simulink model "Battery_ECM"  (R2022b)
settings: Solver=VariableStepAuto  StartTime=0.0  StopTime=30000  RelTol=1e-3
undefined symbols (not defined in the file): C1, C2, eta_charge, eta_discharge, Q_C, R0, R1, R2, SoC0, Ts
settings Model: Creator=Hadi  LastModifiedBy=Hadi

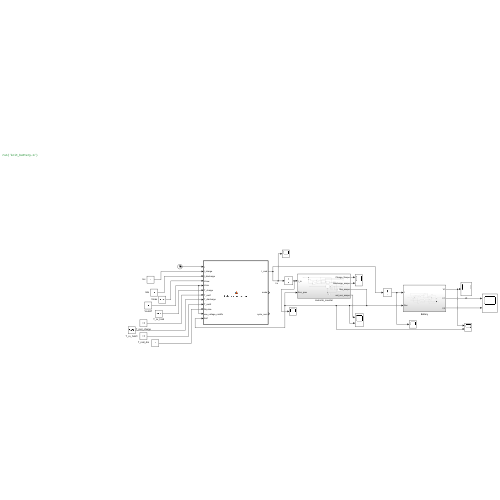
[thumbnail: Simulink's stored preview of the top-level diagram]
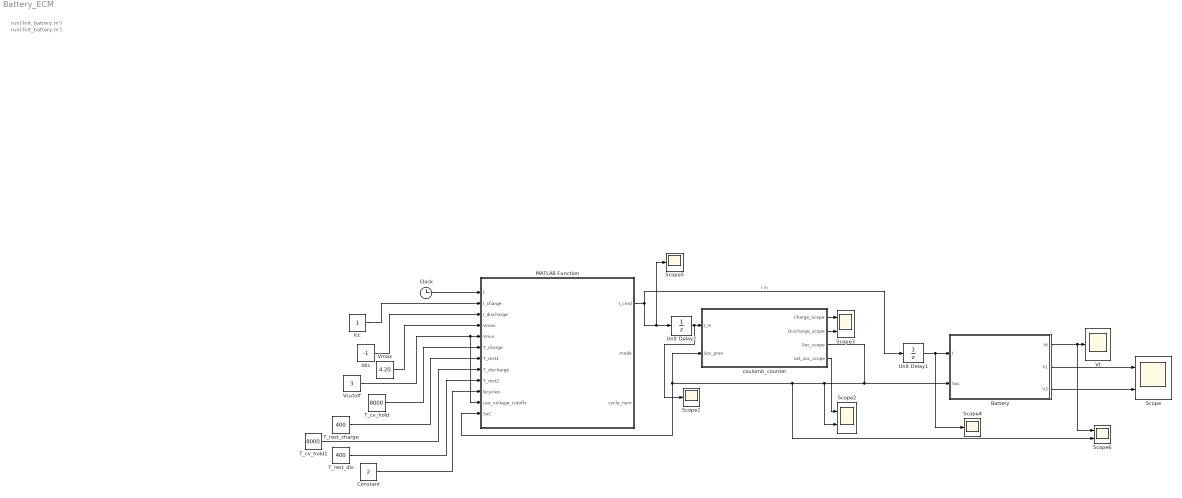
== system Battery_ECM ==
  note: run('init_battery.m')
  note: run('init_battery.m')
  Battery : Subsystem
  Clock : Clock
  Constant : Constant  Value=2
  Icc : Constant
  Idis : Constant  Value=-1
  MATLAB Function : MATLAB Function  TreatAsAtomicUnit=on
  Scope{,2..3,6} (4 alike) : Scope  NumInputPorts=2
  Scope1 : Scope
  Scope4 : Scope
  Scope5 : Scope
  T_cv_hold : Constant  Value=8000
  T_cv_hold1 : Constant  Value=8000
  T_rest_charge : Constant  Value=400
  T_rest_dis : Constant  Value=400
  Unit Delay1 : UnitDelay  SampleTime=0.05  HasFrameUpgradeWarning=on
  Unit Delay2 : UnitDelay  SampleTime=0.05  HasFrameUpgradeWarning=on
  Vcutoff : Constant  Value=3
  Vmax : Constant  Value=4.20
  Vt : Scope
  coulomb_counter : Subsystem
  wires:
  MATLAB Function/1(I_cmd) -> Scope5/1, Unit Delay2/1, Unit Delay1/1  "I in"
  Unit Delay1/1 -> Scope4/1, Battery/1(I)
  coulomb_counter/1(Charge_Scope) -> Scope3/1
  Unit Delay2/1 -> Scope1/1, coulomb_counter/1(I_In)
  coulomb_counter/4(sat_soc_scope) -> Scope2/1
  coulomb_counter/2(Discharge_scope) -> Scope3/2
  coulomb_counter/3(Soc_scope) -> Scope6/2, MATLAB Function/12(SoC), coulomb_counter/2(Soc_prev), Scope2/2, Battery/2(Soc)
  Battery/3(V2) -> Scope/2
  Battery/2(V1) -> Scope/1
  Battery/1(Vt) -> Scope6/1, Vt/1
  Clock/1 -> MATLAB Function/1(t)
  Vmax/1 -> MATLAB Function/4(Vmax)
  Vcutoff/1 -> MATLAB Function/5(Vmin), MATLAB Function/11(use_voltage_cutoffs)
  T_rest_charge/1 -> MATLAB Function/7(T_rest1)
  T_rest_dis/1 -> MATLAB Function/9(T_rest2)
  Icc/1 -> MATLAB Function/2(I_charge)
  Idis/1 -> MATLAB Function/3(I_discharge)
  T_cv_hold/1 -> MATLAB Function/6(T_charge)
  Constant/1 -> MATLAB Function/10(Ncycles)
  T_cv_hold1/1 -> MATLAB Function/8(T_discharge)

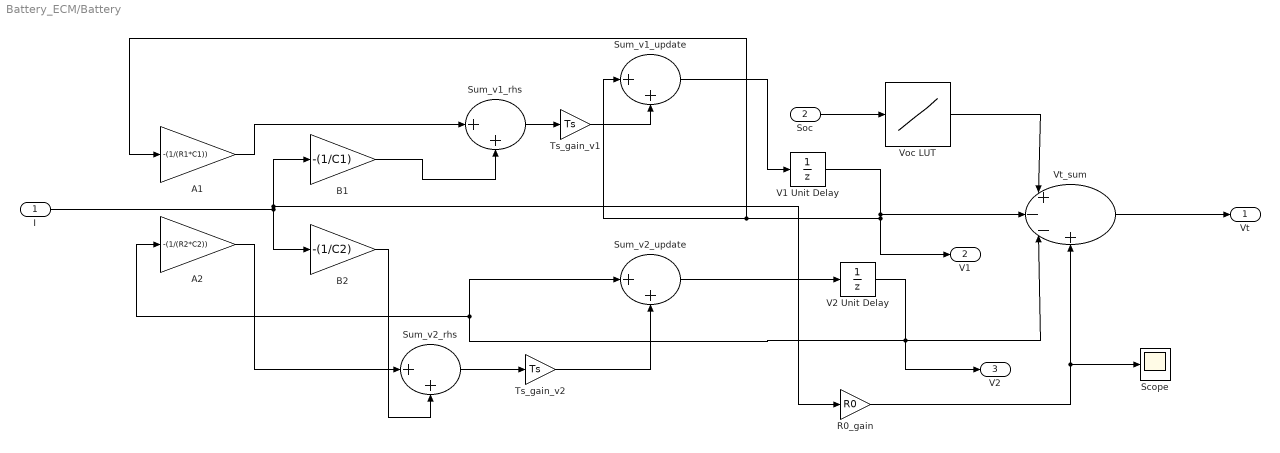
== system Battery_ECM/Battery ==
  I : Inport
  Soc : Inport  Port=2
  A1 : Gain  Gain=-(1/(R1*C1))
  A2 : Gain  Gain=-(1/(R2*C2))
  B1 : Gain  Gain=-(1/C1)
  B2 : Gain  Gain=-(1/C2)
  R0_gain : Gain  Gain=R0
  Scope : Scope
  Sum_v1_rhs : Sum  Inputs=|++
  Sum_v1_update : Sum  Inputs=|++
  Sum_v2_rhs : Sum  Inputs=|++
  Sum_v2_update : Sum  Inputs=|++
  Ts_gain_v1 : Gain  Gain=Ts
  Ts_gain_v2 : Gain  Gain=Ts
  V1 Unit Delay : UnitDelay  SampleTime=-1  HasFrameUpgradeWarning=on
  V2 Unit Delay : UnitDelay  SampleTime=-1  HasFrameUpgradeWarning=on
  Voc LUT : Lookup_n-D  NumberOfTableDimensions=1  BreakpointsForDimension1=[0 0.1 0.2 0.3 0.4 0.5 0.6 0.7 0.8 0.9 1]  Table=[3 3.3 3.5 3.65 3.75 3.85 3.95 4.02 4.07 4.12 4.2]  InternalRulePriority=Speed  RndMeth=Simplest
  Vt_sum : Sum  Inputs=|+--+
  Vt : Outport
  V1 : Outport  Port=2
  V2 : Outport  Port=3
  wires:
  Ts_gain_v2/1 -> Sum_v2_update/2
  I/1 -> B1/1, R0_gain/1, B2/1
  Vt_sum/1 -> Vt/1
  R0_gain/1 -> Scope/1, Vt_sum/4
  V1 Unit Delay/1 -> V1/1, A1/1, Sum_v1_update/1, Vt_sum/2
  V2 Unit Delay/1 -> V2/1, Vt_sum/3, A2/1, Sum_v2_update/1
  A1/1 -> Sum_v1_rhs/1
  Sum_v1_update/1 -> V1 Unit Delay/1
  Sum_v1_rhs/1 -> Ts_gain_v1/1
  Voc LUT/1 -> Vt_sum/1
  Soc/1 -> Voc LUT/1
  Sum_v2_update/1 -> V2 Unit Delay/1
  Sum_v2_rhs/1 -> Ts_gain_v2/1
  Ts_gain_v1/1 -> Sum_v1_update/2
  B1/1 -> Sum_v1_rhs/2
  A2/1 -> Sum_v2_rhs/1
  B2/1 -> Sum_v2_rhs/2

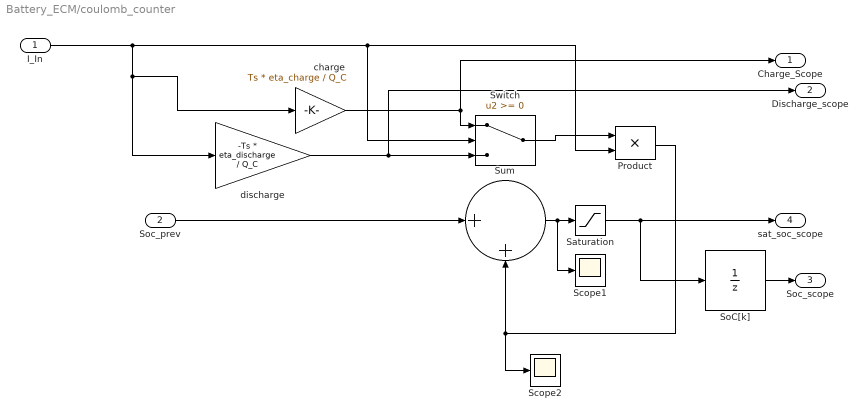
== system Battery_ECM/coulomb_counter ==
  I_In : Inport
  Soc_prev : Inport  Port=2
  Product : Product
  Saturation : Saturate  UpperLimit=1  LowerLimit=0
  Scope1 : Scope
  Scope2 : Scope
  SoC[k] : UnitDelay  InitialCondition=SoC0  SampleTime=-1  HasFrameUpgradeWarning=on
  Sum : Sum  Inputs=|++
  Switch : Switch  SaturateOnIntegerOverflow=off  InputSameDT=off
  charge : Gain  Gain=Ts * eta_charge / Q_C
  discharge : Gain  Gain=-Ts * eta_discharge / Q_C
  Charge_Scope : Outport
  Discharge_scope : Outport  Port=2
  Soc_scope : Outport  Port=3
  sat_soc_scope : Outport  Port=4
  wires:
  charge/1 -> Charge_Scope/1, Switch/1
  Saturation/1 -> SoC[k]/1, sat_soc_scope/1
  Sum/1 -> Scope1/1, Saturation/1
  Switch/1 -> Product/1
  discharge/1 -> Discharge_scope/1, Switch/3
  SoC[k]/1 -> Soc_scope/1
  I_In/1 -> Product/2, Switch/2, discharge/1, charge/1
  Soc_prev/1 -> Sum/1
  Product/1 -> Sum/2, Scope2/1

== matlab function Battery_ECM/MATLAB Function ==
  data: t input; I_charge input; I_discharge input; I_cmd output; Vmax input; Vmin input; T_charge input; T_rest1 input; T_discharge input; T_rest2 input; Ncycles input; use_voltage_cutoffs input; SoC input; mode output; cycle_num output
function [I_cmd, mode, cycle_num] = battery_cycle_control(t, ...
    I_charge, I_discharge, ...
    Vmax, Vmin, ...
    T_charge, T_rest1, T_discharge, T_rest2, ...
    Ncycles, use_voltage_cutoffs, SoC)


I_cmd = 0;
mode = 0;
cycle_num = 0;

if Ncycles < 0
    Ncycles = 0;
end

% One full cycle duration
T_cycle = T_charge + T_rest1 + T_discharge + T_rest2;
if T_cycle <= 0
    return;
end

% compute cycle number and time within cycle
cycle_num = floor(t / T_cycle) + 1;
t_in_cycle = mod(t, T_cycle);

% if we've completed all cycles, idle
if cycle_num > Ncycles
    I_cmd = 0;
    mode = 0;
    return;
end

% Helper: check voltage cutoffs 
if use_voltage_cutoffs ~= 0
    at_charge_cut  = (SoC >= 0.999) || (Vmax <= 0); % fallback if bad Vmax
    at_discharge_cut = (SoC <= 0.001) || (Vmin <= 0);
else
    at_charge_cut = false;
    at_discharge_cut = false;
end

% Choose phase by time-in-cycle, but allow early exits when using voltage cutoffs
if t_in_cycle < T_charge
    % Charge phase (CC)
    % IMPORTANT: I_charge must be passed in as positive. Output I_cmd as positive.
    if use_voltage_cutoffs && (at_charge_cut || (SoC >= 1))
        % If the voltage/SoC cutoff reached early, stop charging and go to rest
        I_cmd = 0;
        mode = 2; % rest after charge
    else
        I_cmd = I_charge; % positive = charging
        mode = 1;
    end

elseif t_in_cycle < (T_charge + T_rest1)
    % Rest after charge
    I_cmd = 0;
    mode = 2;

elseif t_in_cycle < (T_charge + T_rest1 + T_discharge)
    % Discharge phase
    % I_discharge is input as positive magnitude -> function outputs negative current
    if use_voltage_cutoffs && (at_discharge_cut || (SoC <= 0))
        % if Vmin/SoC cutoff reached, stop and go to rest
        I_cmd = 0;
        mode = 4; % rest after discharge
    else
        I_cmd = -abs(I_discharge); % negative = discharging
        mode = 3;
    end

else
    % Rest after discharge
    I_cmd = 0;
    mode = 4;
end

end
